simulink model "pid"  (R2015a)
settings: Solver=ode3  StartTime=0.0  StopTime=10.0  RelTol=1e-3
undefined symbols (not defined in the file): Discovery, LINK, SampleTime, ST, STM32F4
libraries: pil_lib x1
settings Model: Creator=Denis  LastModifiedBy=Denis
settings OptimizationCC: OptimizeModelRefInitCode=on  LifeSpan=1  MaxStackSize=64
settings HardwareCC: ProdLargestAtomicInteger=Long  ProdLargestAtomicFloat=Double  ProdEndianess=LittleEndian  ProdHWDeviceType=ARM Compatible->ARM Cortex
settings RTWCC: SystemTargetFile=ert.tlc  TemplateMakefile=ert_default_tmf  Description=Embedded Coder  Toolchain=GNU Tools for ARM Embedded Processors  CreateSILPILBlock=PIL
settings CodeAppCC: IgnoreCustomStorageClasses=off
settings ERTTargetCC: GenerateSampleERTMain=off  ParMdlRefBuildCompliant=on  CompOptLevelCompliant=on  ConcurrentExecutionCompliant=on  ERTFirstTimeCompliant=on  SupportContinuousTime=off  SupportVariableSizeSignals=off  ModelStepFunctionPrototypeControlCompliant=on  CPPClassGenCompliant=on  InlinedParameterPlacement=Hierarchical

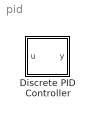
== system pid ==
  Discrete PID Controller : Subsystem  DialogController=pil_create_dialog  LoadFcn=|
      | try
      |    if ~strcmp(rtw.pil.getPILVersion, '6.8 (R2015a)_12')
      |       set_param(gcb, 'DialogController', '');
      |       set_param(gcb, 'DialogControllerArgs', '');
      |    end
      | catch e
      |       set_param(gcb, 'DialogController', '');
      |       set_param(gcb, 'DialogControllerArgs', '');
      | end
      mask help: PIL:pil:XILBlockMaskDesc
      mask Display: disp('PIL');

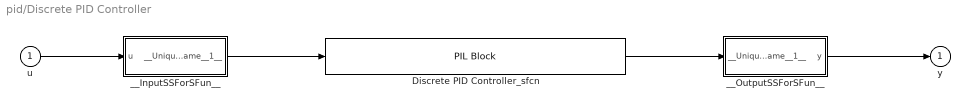
== system pid/Discrete PID Controller ==
  u : Inport
  Discrete PID Controller_sfcn : pil_lib/PIL Block  SimulationMode=PIL  IsTopModelPIL=off  CodeDir=A:\UFCG\TCC\simulink\modelo_servo_pid_1\Discrete_ert_rtw  ConfigName=STM32F4-Discovery (ST-LINK)
  __InputSSForSFun__ : Subsystem
  __OutputSSForSFun__ : Subsystem
  y : Outport  SampleTime=SampleTime  InitialOutput=0
  wires:
  u/1 -> __InputSSForSFun__/1(u)
  __InputSSForSFun__/1(__UniqueOutportName__1__) -> Discrete PID Controller_sfcn/1
  Discrete PID Controller_sfcn/1 -> __OutputSSForSFun__/1(__UniqueInportName__1__)
  __OutputSSForSFun__/1(y) -> y/1

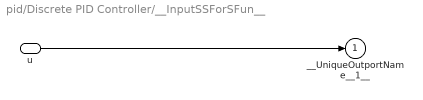
== system pid/Discrete PID Controller/__InputSSForSFun__ ==
  u : Inport
  __UniqueOutportName__1__ : Outport
  wires:
  u/1 -> __UniqueOutportName__1__/1

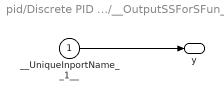
== system pid/Discrete PID Controller/__OutputSSForSFun__ ==
  __UniqueInportName__1__ : Inport
  y : Outport  SampleTime=SampleTime  InitialOutput=0
  wires:
  __UniqueInportName__1__/1 -> y/1
